simulink model "LQGy_sim"  (R2025b)
settings: Solver=ode4  StartTime=0.0  StopTime=T  FixedStep=Ts  RelTol=1e-3
values from neighbouring files (symbols this model uses):
  D = [0 0]'    [IP_MACRO_SIM.m]
  K_i = K_aug(6)    [IP_MACRO_SIM.m]
  K_x = K_aug(1:5)    [IP_MACRO_SIM.m]
  L = lqe(A, G, C, Qe, Re)    [IP_MACRO_SIM.m]
  x0 = [0.3 -2 0.4 1 0]'    [IP_MACRO_SIM.m]
undefined symbols (not defined in the file or in its folder): A, B, C
settings Model: Creator=leita  LastModifiedBy=Asus
settings DataIOCC: ReturnWorkspaceOutputs=off

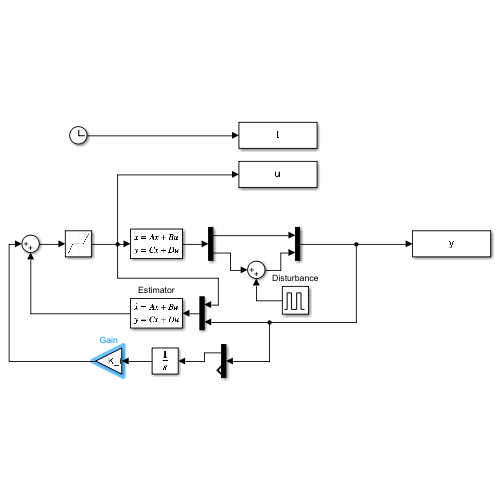
[thumbnail: Simulink's stored preview of the top-level diagram]
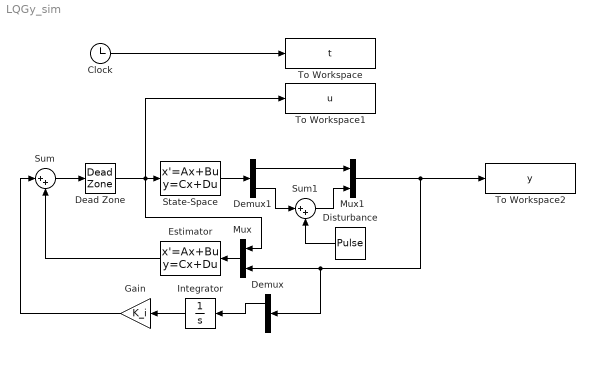
== system LQGy_sim ==
  Clock : Clock
  Dead Zone : DeadZone  LowerValue=-0.2  UpperValue=0.2
  Demux : Demux  Outputs=2
  Demux1 : Demux  Outputs=2
  Disturbance : DiscretePulseGenerator  PulseType=Time based  Amplitude=0.12  PulseWidth=5
  Estimator : StateSpace  A=A-L*C  B=[B, L]  C=-K_x  D=zeros(1, 1 + size(C, 1))  InitialCondition=0
  Gain : Gain  Gain=K_i
  Integrator : Integrator
  Mux : Mux  Inputs=2
  Mux1 : Mux  Inputs=2
  State-Space : StateSpace  A=A  B=B  C=C  D=D  InitialCondition=x0
  Sum : Sum  Inputs=|++
  Sum1 : Sum  Inputs=|++
  To Workspace : ToWorkspace  VariableName=t  SaveFormat=Timeseries  SampleTime=-1
  To Workspace1 : ToWorkspace  VariableName=u  SaveFormat=Timeseries  SampleTime=-1
  To Workspace2 : ToWorkspace  VariableName=y  SaveFormat=Timeseries  SampleTime=-1
  wires:
  Clock/1 -> To Workspace/1
  Mux/1 -> Estimator/1
  Sum/1 -> Dead Zone/1
  Estimator/1 -> Sum/2
  Demux/1 -> Integrator/1
  Integrator/1 -> Gain/1
  Gain/1 -> Sum/1
  Dead Zone/1 -> Mux/1, To Workspace1/1, State-Space/1
  Demux1/1 -> Mux1/1
  State-Space/1 -> Demux1/1
  Mux1/1 -> Demux/1, Mux/2, To Workspace2/1
  Sum1/1 -> Mux1/2
  Demux1/2 -> Sum1/1
  Disturbance/1 -> Sum1/2
